simulink model "Michaela_Model_Attempt_3"  (R2020a)
settings: Solver=VariableStepAuto  StartTime=0.0  StopTime=0.02  RelTol=1e-3
libraries: fl_lib x18, nesl_utility x5, ee_lib x4
settings Model: Creator=mgfee  LastModifiedBy=mgfee

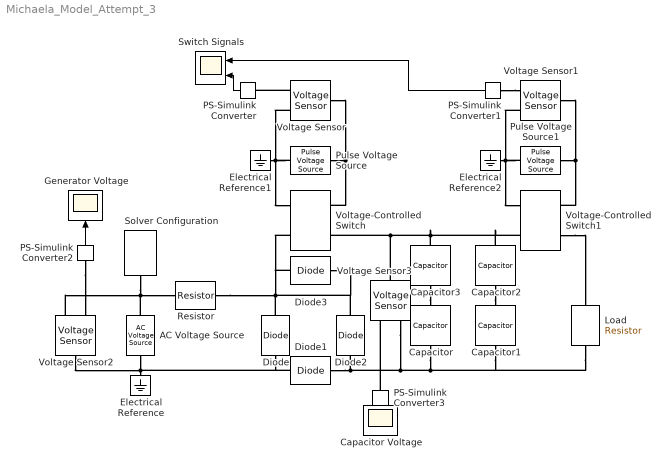
== system Michaela_Model_Attempt_3 ==
  AC Voltage Source : fl_lib/Electrical/Electrical Sources/AC Voltage Source  amp=20 V  shift=0 deg  frequency=60 Hz  omega=0 rad/s
  Capacitor{,1..3} (4 alike) : fl_lib/Electrical/Electrical Elements/Capacitor  c=1 F  r=1e-6 Ohm  g=0 1/Ohm  i_specify=off  i_priority=None  i=0 A  i_nominal_specify=off  i_nominal_unit=A  i_nominal_value=1  v_specify=off  v_priority=None  v=0 V  v_nominal_specify=off  v_nominal_unit=V  v_nominal_value=1  vc_specify=off  vc_priority=High  vc=0 V  vc_nominal_specify=off  vc_nominal_unit=V  vc_nominal_value=1
  Capacitor Voltage : Scope
  Diode{,1..3} (4 alike) : fl_lib/Electrical/Electrical Elements/Diode  Vf=0.6 V  Ron=0.3 Ohm  Goff=1e-8 1/Ohm  i_specify=off  i_priority=None  i=0 A  i_nominal_specify=off  i_nominal_unit=A  i_nominal_value=1  v_specify=off  v_priority=None  v=0 V  v_nominal_specify=off  v_nominal_unit=V  v_nominal_value=1
  Electrical Reference : fl_lib/Electrical/Electrical Elements/Electrical Reference
  Electrical Reference1 : fl_lib/Electrical/Electrical Elements/Electrical Reference
  Electrical Reference2 : fl_lib/Electrical/Electrical Elements/Electrical Reference
  Generator Voltage : Scope
  Load : fl_lib/Electrical/Electrical Elements/Resistor  R=0.1 Ohm  i_specify=off  i_priority=None  i=0 A  i_nominal_specify=off  i_nominal_unit=A  i_nominal_value=1  v_specify=off  v_priority=None  v=0 V  v_nominal_specify=off  v_nominal_unit=V  v_nominal_value=1
  PS-Simulink Converter{,1..3} (4 alike) : nesl_utility/PS-Simulink Converter  PhysicalDomain=network_engine_domain  SubClassName=ps_output  LeftPortType=input  RightPortType=output  PseudoPeriodic=off  Frequencies=[]  Unit=inherit  AffineConversion=off
  Pulse Voltage Source : ee_lib/Additional Components/SPICE Sources/Pulse Voltage Source  V1=0 V  V2=1 V  TD=0 s  TR=1e-9 s  TF=1e-9 s  PW=5 ms  PER=10 ms
      settings: SourceProductBaseCode=PS  InternalSimscapePortConfiguration="{\"Bottom\":[],\"Left\":[{\"id\":\"p\",\"label\":\"\",\"type\":\"foundation.electrical.electrical\"}],\"Right\":[{\"id\":\"n\",\"label\":\"\",\"type\":\"foundation.electrical.electrical\"}],\"Top\":[]}"
  Pulse Voltage Source1 : ee_lib/Additional Components/SPICE Sources/Pulse Voltage Source  V1=0 V  V2=1 V  TD=5 ms  TR=1e-9 s  TF=1e-9 s  PW=1 ms  PER=10 ms
      settings: SourceProductBaseCode=PS  InternalSimscapePortConfiguration="{\"Bottom\":[],\"Left\":[{\"id\":\"p\",\"label\":\"\",\"type\":\"foundation.electrical.electrical\"}],\"Right\":[{\"id\":\"n\",\"label\":\"\",\"type\":\"foundation.electrical.electrical\"}],\"Top\":[]}"
  Resistor : fl_lib/Electrical/Electrical Elements/Resistor  R=10 Ohm  i_specify=off  i_priority=None  i=0 A  i_nominal_specify=off  i_nominal_unit=A  i_nominal_value=1  v_specify=off  v_priority=None  v=0 V  v_nominal_specify=off  v_nominal_unit=V  v_nominal_value=1
  Solver Configuration : nesl_utility/Solver Configuration  PhysicalDomain=network_engine_domain  SubClassName=solver  LeftPortType=input  RightPortType=generic  Tones=[]  Harmonics=[]  SimulateNoise=off  Profile=off  UseLocalSampling=off  EnableSwitchedLinearOptims=on  FrequencyDomain=off  UseCCode=off  RelTol=0.001  AbsTol=1e-06  MinStep=1e-09  ToWorkspace=off  RevertToSquareIcSolve=off  NumHomotopyIterations=100  PhasorMode=off  PhasorModeNumHarmonics=1  DoDC=off  ResidualTolerance=1e-09  UseLocalSolver=off  LocalSolverChoice=NE_BACKWARD_EULER_ADVANCER  LocalSolverSampleTime=0.001  DoFixedCost=off  MaxNonlinIter=3  MaxModeIter=2  LinearAlgebra=auto  EquationFormulation=NE_TIME_EF  DelaysMemoryBudget=1024  AutomaticFiltering=on  FilteringTimeConstant=0.001  PartitionStorageMethod=AS_NEEDED  PartitionMemoryBudget=1024  PartitionMethod=ROBUST
  Switch Signals : Scope  NumInputPorts=2
  Voltage Sensor{,1..3} (4 alike) : fl_lib/Electrical/Electrical Sensors/Voltage Sensor
  Voltage-Controlled Switch : ee_lib/Additional Components/SPICE Passives/Voltage-Controlled Switch  VT=0 V  VH=0 V  RON=1 Ohm  ROFF=1e12 Ohm  IC_state=1
      settings: SourceProductBaseCode=PS  InternalSimscapePortConfiguration="{\"Bottom\":[],\"Left\":[{\"id\":\"p1\",\"label\":\"1+\",\"type\":\"foundation.electrical.electrical\"},{\"id\":\"p2\",\"label\":\"2+\",\"type\":\"foundation.electrical.electrical\"}],\"Right\":[{\"id\":\"n1\",\"label\":\"1-\",\"type\":\"foundation.electrical.electrical\"},{\"id\":\"n2\",\"label\":\"2-\",\"type\":\"foundation.electrical.electrical\"}],\"Top\":[]}"
  Voltage-Controlled Switch1 : ee_lib/Additional Components/SPICE Passives/Voltage-Controlled Switch  VT=0 V  VH=0 V  RON=1 Ohm  ROFF=1e12 Ohm  IC_state=1
      settings: SourceProductBaseCode=PS  InternalSimscapePortConfiguration="{\"Bottom\":[],\"Left\":[{\"id\":\"p1\",\"label\":\"1+\",\"type\":\"foundation.electrical.electrical\"},{\"id\":\"p2\",\"label\":\"2+\",\"type\":\"foundation.electrical.electrical\"}],\"Right\":[{\"id\":\"n1\",\"label\":\"1-\",\"type\":\"foundation.electrical.electrical\"},{\"id\":\"n2\",\"label\":\"2-\",\"type\":\"foundation.electrical.electrical\"}],\"Top\":[]}"
  wires:
  PS-Simulink Converter1/1 -> Switch Signals/1
  PS-Simulink Converter/1 -> Switch Signals/2
  PS-Simulink Converter2/1 -> Generator Voltage/1
  connections:
  AC Voltage Source/LConn1 -- Voltage Sensor2/RConn2 -- Solver Configuration/RConn1 -- Resistor/LConn1
  AC Voltage Source/RConn1 -- Voltage Sensor2/LConn1 -- Diode/LConn1 -- Diode1/RConn1 -- Electrical Reference/LConn1
  Diode1/LConn1 -- Load/RConn1 -- Capacitor1/RConn1 -- Capacitor/RConn1 -- Voltage Sensor3/RConn2 -- Diode2/LConn1
  Resistor/RConn1 -- Voltage-Controlled Switch/RConn2 -- Diode3/RConn1 -- Diode3/LConn1 -- Diode2/RConn1 -- Diode/RConn1
  Capacitor2/RConn1 -- Capacitor1/LConn1
  Capacitor3/RConn1 -- Capacitor/LConn1
  Voltage-Controlled Switch1/RConn2 -- Capacitor2/LConn1 -- Capacitor3/LConn1 -- Voltage Sensor3/LConn1 -- Voltage-Controlled Switch/LConn2
  Voltage-Controlled Switch1/LConn2 -- Load/LConn1
  Pulse Voltage Source/LConn1 -- Voltage Sensor/LConn1 -- Voltage-Controlled Switch/LConn1
  Pulse Voltage Source1/LConn1 -- Voltage Sensor1/LConn1 -- Voltage-Controlled Switch1/LConn1
  Pulse Voltage Source1/RConn1 -- Voltage Sensor1/RConn2 -- Electrical Reference2/LConn1 -- Voltage-Controlled Switch1/RConn1
  Pulse Voltage Source/RConn1 -- Voltage Sensor/RConn2 -- Electrical Reference1/LConn1 -- Voltage-Controlled Switch/RConn1
  Voltage Sensor/RConn1 -- PS-Simulink Converter/LConn1
  PS-Simulink Converter1/LConn1 -- Voltage Sensor1/RConn1
  PS-Simulink Converter2/LConn1 -- Voltage Sensor2/RConn1
  PS-Simulink Converter3/LConn1 -- Voltage Sensor3/RConn1
